simulink model "untitled"  (R2020a)
settings: Solver=VariableStepAuto  StartTime=0.0  StopTime=10.0  RelTol=1e-3
libraries: simulink x1
settings Model: Creator=jambox  LastModifiedBy=jambox

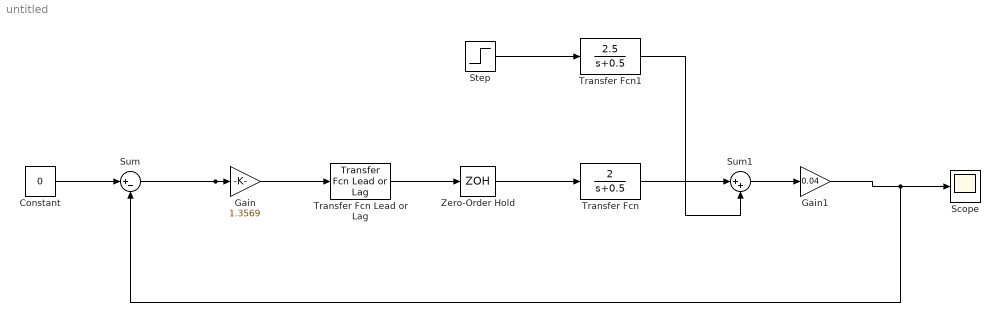
== system untitled ==
  Constant : Constant  Value=0
  Gain : Gain  Gain=1.3569
  Gain1 : Gain  Gain=0.04
  Scope : Scope
  Step : Step  SampleTime=0
  Sum : Sum  Inputs=|+-
  Sum1 : Sum  Inputs=|++
  Transfer Fcn : TransferFcn  Numerator=[2]  Denominator=[1 0.5]
  Transfer Fcn Lead or Lag : simulink/Discrete/Transfer Fcn Lead or Lag  PoleZ=0.5488  ZeroZ=0.002479  ICPrevOutput=0.0  ICPrevInput=0.0  DoSatur=off
      settings: SourceProductBaseCode=SL
  Transfer Fcn1 : TransferFcn  Numerator=2.5  Denominator=[1 0.5]
  Zero-Order Hold : ZeroOrderHold  SampleTime=-1
  wires:
  Constant/1 -> Sum/1
  Sum/1 -> Gain/1
  Gain/1 -> Transfer Fcn Lead or Lag/1
  Transfer Fcn Lead or Lag/1 -> Zero-Order Hold/1
  Zero-Order Hold/1 -> Transfer Fcn/1
  Step/1 -> Transfer Fcn1/1
  Transfer Fcn1/1 -> Sum1/2
  Transfer Fcn/1 -> Sum1/1
  Gain1/1 -> Sum/2, Scope/1
  Sum1/1 -> Gain1/1
